simulink model "FinalProjectKFSim"  (R2020a)
settings: Solver=VariableStepAuto  StartTime=0.0  StopTime=15  RelTol=1e-3
undefined symbols (not defined in the file): F, H, Q, R
settings Model: Creator=Frab  LastModifiedBy=Frab

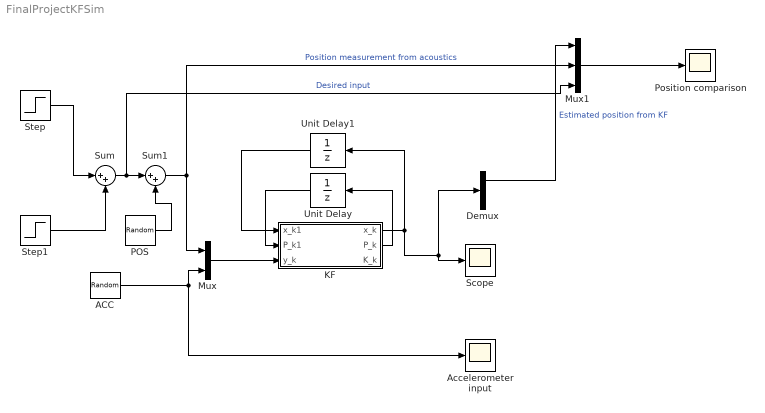
== system FinalProjectKFSim ==
  ACC : RandomNumber  Mean=100  Variance=13.82  SampleTime=0.1
  Accelerometer input : Scope
  Demux : Demux  Outputs=3
  KF : Subsystem
  Mux : Mux  Inputs=2
  Mux1 : Mux  Inputs=3
  POS : RandomNumber  Variance=39.61  SampleTime=.1
  Position comparison : Scope
  Scope : Scope
  Step : Step  After=50  SampleTime=0
  Step1 : Step  Time=5  After=-25  SampleTime=0
  Sum : Sum  Inputs=|++
  Sum1 : Sum  Inputs=|++
  Unit Delay : UnitDelay  InitialCondition=eye(3)  SampleTime=-1  HasFrameUpgradeWarning=on
  Unit Delay1 : UnitDelay  InitialCondition=[0; 0; 0]  SampleTime=-1  HasFrameUpgradeWarning=on
  wires:
  ACC/1 -> Accelerometer input/1, Mux/2
  Mux/1 -> KF/3(y_k)
  KF/1(x_k) -> Demux/1, Scope/1, Unit Delay1/1
  KF/2(P_k) -> Unit Delay/1
  Unit Delay/1 -> KF/2(P_k1)
  Unit Delay1/1 -> KF/1(x_k1)
  Step/1 -> Sum/1
  Demux/1 -> Mux1/1  "Estimated position from KF"
  Mux1/1 -> Position comparison/1
  Sum/1 -> Mux1/3, Sum1/1  "Desired input"
  POS/1 -> Sum1/2
  Step1/1 -> Sum/2
  Sum1/1 -> Mux/1, Mux1/2  "Position measurement from acoustics"

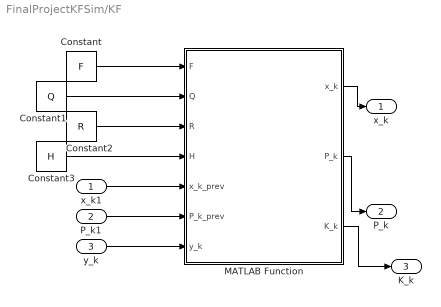
== system FinalProjectKFSim/KF ==
  x_k1 : Inport
  P_k1 : Inport  Port=2
  y_k : Inport  Port=3
  Constant : Constant  Value=F  VectorParams1D=off
  Constant1 : Constant  Value=Q  VectorParams1D=off
  Constant2 : Constant  Value=R  VectorParams1D=off
  Constant3 : Constant  Value=H  VectorParams1D=off
  MATLAB Function : MATLAB Function  TreatAsAtomicUnit=on
  x_k : Outport
  P_k : Outport  Port=2
  K_k : Outport  Port=3
  wires:
  x_k1/1 -> MATLAB Function/5(x_k_prev)
  P_k1/1 -> MATLAB Function/6(P_k_prev)
  y_k/1 -> MATLAB Function/7(y_k)
  MATLAB Function/2(P_k) -> P_k/1
  MATLAB Function/1(x_k) -> x_k/1
  Constant3/1 -> MATLAB Function/4(H)
  Constant2/1 -> MATLAB Function/3(R)
  Constant1/1 -> MATLAB Function/2(Q)
  Constant/1 -> MATLAB Function/1(F)
  MATLAB Function/3(K_k) -> K_k/1

== matlab function FinalProjectKFSim/KF/MATLAB Function ==
  data: F input; x_k output; Q input; R input; H input; x_k_prev input; P_k_prev input; y_k input; P_k output; K_k output
function [x_k, P_k, K_k] = KF(F, Q, R, H, x_k_prev, P_k_prev, y_k)
    x_k_m = F * x_k_prev;
    P_k_m = F * P_k_prev * (F') + Q;
    
    W_k = H * P_k_m * (H') + R;
    K_k = P_k_m * (H') * (W_k)^(-1);
    y_k_m = H * x_k_m;
    x_k = x_k_m + K_k * (y_k - y_k_m);
    P_k = P_k_m - K_k * H * P_k_m - P_k_m * (H') * (K_k') + K_k * W_k * (K_k');

end
